simulink model "Kalman"  (R2023b)
settings: Solver=VariableStepAuto  StartTime=0.0  StopTime=200  RelTol=1e-3
values from neighbouring files (symbols this model uses):
  Tm2 = 3    [Lab3.m]
  Ts2 = Tm2/5    (= 0.6)    [Lab3.m]
undefined symbols (not defined in the file or in its folder): denF, denR, denR2, denR4, numF, numR, numR2, numR4
settings Model: Creator=raluc  LastModifiedBy=raluc

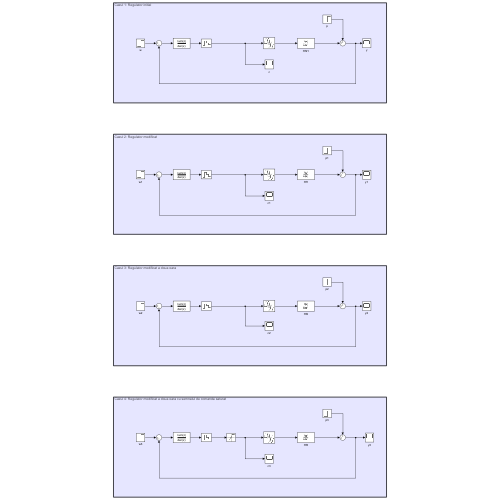
[thumbnail: Simulink's stored preview of the top-level diagram]
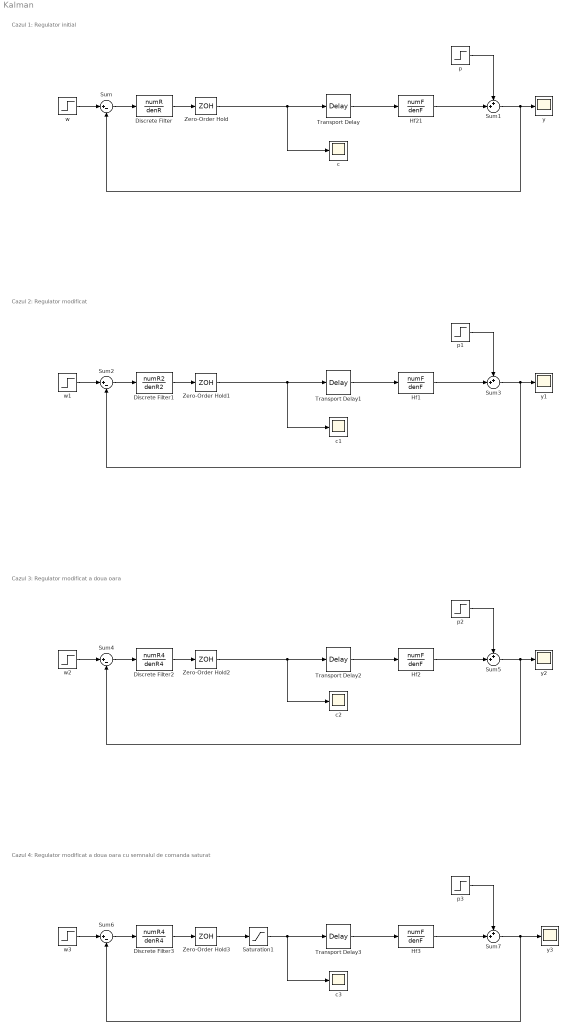
== system Kalman ==
  note: Cazul 1: Regulator initial
  note: Cazul 2: Regulator modificat
  note: Cazul 3: Regulator modificat a doua oara
  note: Cazul 4: Regulator modificat a doua oara cu semnalul de comanda saturat
  Discrete Filter : DiscreteFilter  Numerator=numR  Denominator=denR
  Discrete Filter1 : DiscreteFilter  Numerator=numR2  Denominator=denR2
  Discrete Filter2 : DiscreteFilter  Numerator=numR4  Denominator=denR4
  Discrete Filter3 : DiscreteFilter  Numerator=numR4  Denominator=denR4
  Hf{1..3,21} (4 alike) : TransferFcn  Numerator=numF  Denominator=denF
  Saturation1 : Saturate  UpperLimit=1  LowerLimit=0.
  Sum{,2,4,6} (4 alike) : Sum  Inputs=|+-
  Sum{1,3,5,7} (4 alike) : Sum  Inputs=++|
  Transport Delay{,1..3} (4 alike) : TransportDelay  DelayTime=Tm2
  Zero-Order Hold{,1..3} (4 alike) : ZeroOrderHold  SampleTime=Ts2
  c{,1..3} (4 alike) : Scope
  p{,1..3} (4 alike) : Step  After=0  SampleTime=0
  w{,1..3} (4 alike) : Step  SampleTime=0
  y{,1..3} (4 alike) : Scope
  wires:
  Sum/1 -> Discrete Filter/1
  Discrete Filter/1 -> Zero-Order Hold/1
  Sum1/1 -> Sum/2, y/1
  Hf21/1 -> Sum1/2
  p/1 -> Sum1/1
  w/1 -> Sum/1
  Transport Delay/1 -> Hf21/1
  Zero-Order Hold/1 -> c/1, Transport Delay/1
  Sum3/1 -> y1/1, Sum2/2
  p1/1 -> Sum3/1
  Hf1/1 -> Sum3/2
  Transport Delay1/1 -> Hf1/1
  Discrete Filter1/1 -> Zero-Order Hold1/1
  w1/1 -> Sum2/1
  Sum2/1 -> Discrete Filter1/1
  Zero-Order Hold1/1 -> c1/1, Transport Delay1/1
  Sum5/1 -> y2/1, Sum4/2
  p2/1 -> Sum5/1
  Hf2/1 -> Sum5/2
  Transport Delay2/1 -> Hf2/1
  Discrete Filter2/1 -> Zero-Order Hold2/1
  w2/1 -> Sum4/1
  Sum4/1 -> Discrete Filter2/1
  Zero-Order Hold2/1 -> c2/1, Transport Delay2/1
  w3/1 -> Sum6/1
  Saturation1/1 -> c3/1, Transport Delay3/1
  Sum6/1 -> Discrete Filter3/1
  Sum7/1 -> y3/1, Sum6/2
  Hf3/1 -> Sum7/2
  Discrete Filter3/1 -> Zero-Order Hold3/1
  Transport Delay3/1 -> Hf3/1
  Zero-Order Hold3/1 -> Saturation1/1
  p3/1 -> Sum7/1
